simulink library "GPS_processing_lib"  (R2016b)
settings: Solver=VariableStepAuto  StartTime=0.0  StopTime=10.0  RelTol=1e-3
libraries: eci_2_TLE_lib x1
settings Model: Creator=taylorreynolds  LastModifiedBy=Taylor

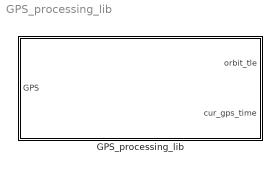
== system GPS_processing_lib ==
  GPS_processing_lib : Subsystem

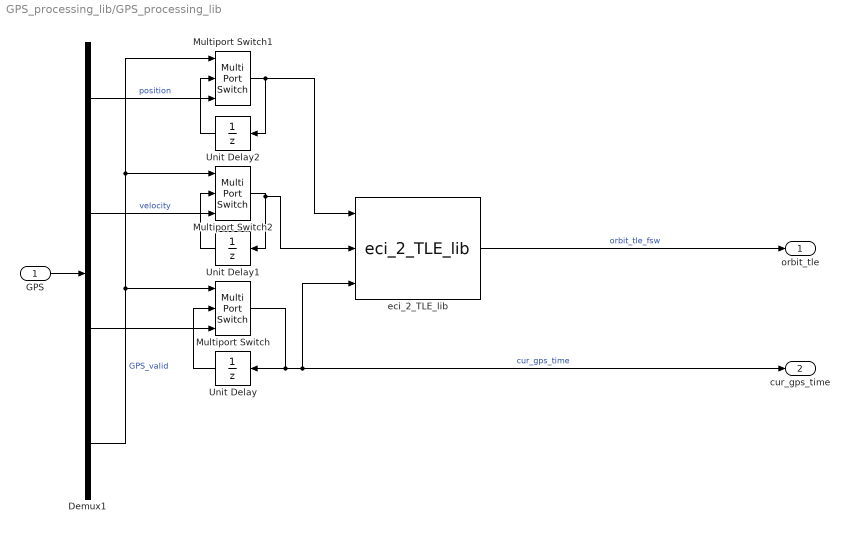
== system GPS_processing_lib/GPS_processing_lib ==
  GPS : Inport
  Demux1 : Demux  Outputs=[3 3 2 1]
  Multiport Switch : MultiPortSwitch  DataPortOrder=Zero-based contiguous  Inputs=2
  Multiport Switch1 : MultiPortSwitch  DataPortOrder=Zero-based contiguous  Inputs=2
  Multiport Switch2 : MultiPortSwitch  DataPortOrder=Zero-based contiguous  Inputs=2
  Unit Delay : UnitDelay  InitialCondition=fsw_params.sensor_processing.gps.ic.time  SampleTime=-1
  Unit Delay1 : UnitDelay  InitialCondition=fsw_params.sensor_processing.gps.ic.vel  SampleTime=-1
  Unit Delay2 : UnitDelay  InitialCondition=fsw_params.sensor_processing.gps.ic.pos  SampleTime=-1
  eci_2_TLE_lib : eci_2_TLE_lib/eci_2_TLE_lib
  orbit_tle : Outport
  cur_gps_time : Outport  Port=2
  wires:
  Multiport Switch2/1 -> Unit Delay1/1, eci_2_TLE_lib/2
  Multiport Switch1/1 -> Unit Delay2/1, eci_2_TLE_lib/1
  Unit Delay2/1 -> Multiport Switch1/2
  Unit Delay1/1 -> Multiport Switch2/2
  GPS/1 -> Demux1/1
  Demux1/1 -> Multiport Switch1/3  "position"
  Demux1/2 -> Multiport Switch2/3  "velocity"
  Demux1/3 -> Multiport Switch/3
  eci_2_TLE_lib/1 -> orbit_tle/1  "orbit_tle_fsw"
  Multiport Switch/1 -> Unit Delay/1, cur_gps_time/1, eci_2_TLE_lib/3  "cur_gps_time"
  Unit Delay/1 -> Multiport Switch/2
  Demux1/4 -> Multiport Switch/1, Multiport Switch2/1, Multiport Switch1/1  "GPS_valid"
